simulink model "duffing"  (R2021a)
settings: Solver=FixedStepAuto  StartTime=0.0  StopTime=10.0  RelTol=1e-3
libraries: simulink x1
settings Model: Creator=surya  LastModifiedBy=surya
settings RTWCC: GenerateReport=on  LaunchReport=on

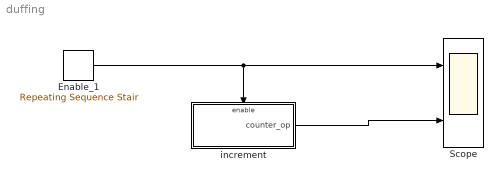
== system duffing ==
  Enable_1 : simulink/Sources/Repeating Sequence Stair  OutValues=[0 1 0 1 1].'  tsamp=-1  OutMin=[]  OutMax=[]  OutDataTypeStr=double  OutputDataTypeScalingMode=double  OutDataType=fixdt(0,8)  ConRadixGroup=Best Precision: Vector-wise  OutScaling=2^-12
  Scope : Scope  NumInputPorts=2
  increment : Subsystem  TreatAsAtomicUnit=on
  wires:
  Enable_1/1 -> Scope/1, increment/Enable
  increment/1(counter_op) -> Scope/2

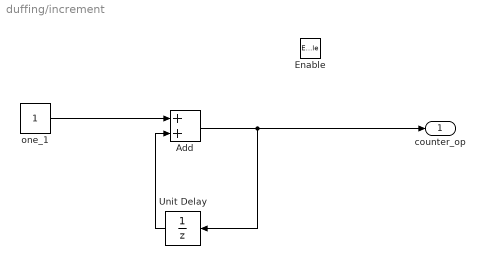
== system duffing/increment ==
  Enable : EnablePort
  Add : Sum
  Unit Delay : UnitDelay  SampleTime=-1  HasFrameUpgradeWarning=on
  one_1 : Constant
  counter_op : Outport
  wires:
  Add/1 -> Unit Delay/1, counter_op/1
  Unit Delay/1 -> Add/2
  one_1/1 -> Add/1
